simulink model "verify_Fuel_CONF_mdl"  (R2016b)
settings: Solver=VariableStepDiscrete  StartTime=0  StopTime=1  MaxStep=1  RelTol=1e-3  EnableMultiTasking=on
InitFcn:
  | load('DE_TRY2010_13_averageYear')
undefined symbols (not defined in the file or in its folder): path_carnot
libraries: carnot x1
settings Model: Creator=drhf  LastModifiedBy=drhf
settings DataIOCC: SaveFormat=Array  SignalLoggingSaveFormat=ModelDataLogs
settings OptimizationCC: ExpressionDepthLimit=2147483647  LifeSpan=inf
settings DebuggingCC: UnderspecifiedInitializationDetection=Classic  MergeDetectMultiDrivingBlocksExec=none  SolverPrmCheckMsg=warning  FcnCallInpInsideContextMsg=warning  StateNameClashWarn=warning  SFUnexpectedBacktrackingDiag=warning  SFNoUnconditionalDefaultTransitionDiag=warning  SFExecutionAtInitializationDiag=none
settings HardwareCC: ProdBitPerPointer=32  ProdBitPerSizeT=32  ProdBitPerPtrDiffT=32  ProdLargestAtomicFloat=None  ProdIntDivRoundTo=Undefined  ProdEndianess=Unspecified  ProdWordSize=32  ProdHWDeviceType=32-bit Generic
settings ModelReferenceCC: PropagateSignalLabelsOutOfModel=off
settings GRTTargetCC: TargetLangStandard=C89/C90 (ANSI)  GeneratePreprocessorConditionals=Disable all  CombineOutputUpdateFcns=off  GRTInterface=on
settings ConfigComp: CovMetricSettings=dw  CovHtmlReporting=on  CovSaveCumulativeToWorkspaceVar=on  CovSaveSingleToWorkspaceVar=on  CovExternalEMLEnable=off

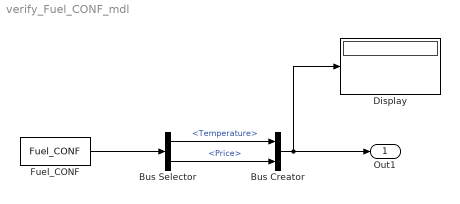
== system verify_Fuel_CONF_mdl ==
  Bus Creator : BusCreator  Inputs=2
  Bus Selector : BusSelector  OutputSignals=Temperature,Price
  Display : Display
  Fuel_CONF : carnot/Source/Energy/Fuel_CONF  Temperature=20  Pressure=101300  PathName=fullfile(path_carnot('libsl'), 'Source','Energy','Fuel_CONF','parameter_set')  FileName='DefaultFuel_Gas.mat'  userPath=off  userParam=off  ft=1  stoichAir=3.5  combustion_enthalpy=[51400000 56900000]  Tcondensation=[45 25]  massfraction=[0.33 0.67 0 0 0 0]  price=1
  Out1 : Outport
  wires:
  Bus Creator/1 -> Display/1, Out1/1
  Fuel_CONF/1 -> Bus Selector/1
  Bus Selector/2 -> Bus Creator/2  "<Price>"
  Bus Selector/1 -> Bus Creator/1  "<Temperature>"
